simulink model "Computer_Side"  (Simulink 10.0)
settings: Solver=VariableStepAuto  StartTime=0.0  StopTime=inf  FixedStep=1  RelTol=1e-3
undefined symbols (not defined in the file): serial
libraries: instrumentlib x3
settings Model: Creator=fredd  LastModifiedBy=fredd
settings DataIOCC: SaveFormat=Dataset  ReturnWorkspaceOutputs=on
settings OptimizationCC: LifeSpan=auto
settings DebuggingCC: UnderspecifiedInitializationDetection=Simplified  MergeDetectMultiDrivingBlocksExec=error  SFUnexpectedBacktrackingDiag=error  SFNoUnconditionalDefaultTransitionDiag=error  SFExecutionAtInitializationDiag=warning  ArithmeticOperatorsInVariantConditions=error
settings HardwareCC: ProdBitPerPointer=64  ProdBitPerSizeT=64  ProdBitPerPtrDiffT=64  ProdLargestAtomicFloat=Float  ProdIntDivRoundTo=Zero  ProdEndianess=LittleEndian  ProdWordSize=64  ProdHWDeviceType=Intel->x86-64 (Windows64)
settings ModelReferenceCC: PropagateSignalLabelsOutOfModel=on
settings SFSimCC: SimUseLocalCustomCode=on  CustomCodeUndefinedFunction=FilterOut
settings RTWCC: RTWUseLocalCustomCode=on
settings CodeAppCC: StateflowObjectComments=off
settings GRTTargetCC: TargetLangStandard=C99 (ISO)  CombineOutputUpdateFcns=on  GRTInterface=off
settings ConfigComp: CovMetricSettings=dwe  CovHtmlReporting=off  CovSaveCumulativeToWorkspaceVar=off  CovSaveSingleToWorkspaceVar=off

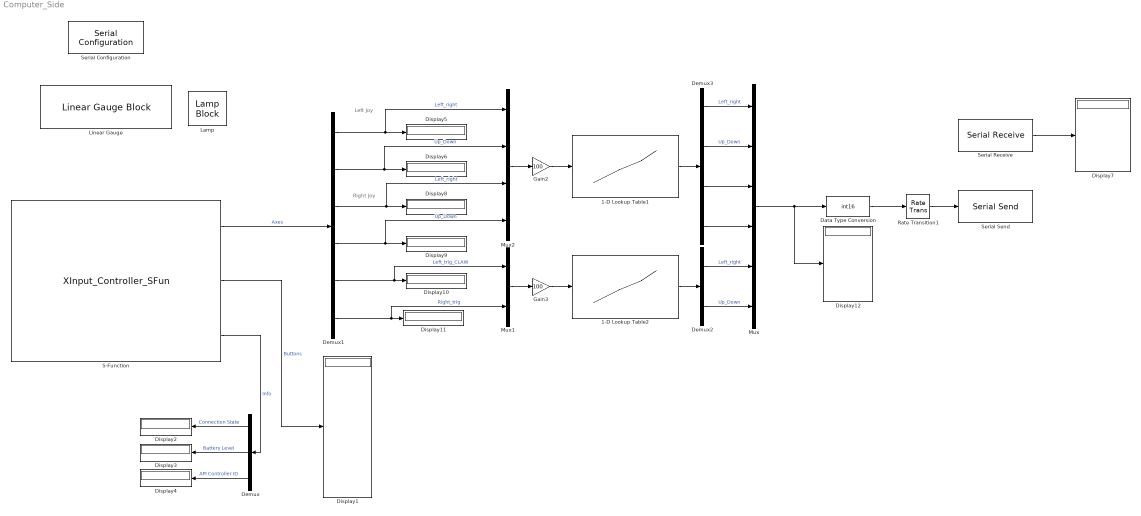
== system Computer_Side ==
  note: Left Joy
  note: Right Joy
  1-D Lookup Table1 : Lookup_n-D  NumberOfTableDimensions=1  BreakpointsForDimension1=[-100,-50,0,50,100]  BreakpointsForDimension1FirstPoint=0  BreakpointsForDimension1Spacing=1.8  Table=[0;45;90;135;180]  InternalRulePriority=Speed  RndMeth=Simplest  InputSameDT=on
  1-D Lookup Table2 : Lookup_n-D  NumberOfTableDimensions=1  BreakpointsForDimension1=[0:5:100]  BreakpointsForDimension1FirstPoint=0  BreakpointsForDimension1Spacing=1.8  Table=[0;9;18;27;36;45;54;63;72;81;90;99;108;117;126;135;144;153;162;171;180]  InternalRulePriority=Speed  RndMeth=Simplest  InputSameDT=on
  Data Type Conversion : DataTypeConversion  OutMin=0  OutMax=100  OutDataTypeStr=int16  RndMeth=Round  SaturateOnIntegerOverflow=on
  Demux : Demux  Outputs=3
  Demux1 : Demux  Outputs=6
  Demux2 : Demux  Outputs=2
  Demux3 : Demux
  Display{1..12} (12 alike) : Display
      Display10 settings: Format=bank  Decimation=2
      Display11 settings: Format=bank  Decimation=2
      Display12 settings: Format=bank  Decimation=2
      Display5 settings: Format=bank  Decimation=2
      Display6 settings: Format=bank  Decimation=2
      Display7 settings: Format=bank  Decimation=2
      Display8 settings: Format=bank  Decimation=2
      Display9 settings: Format=bank  Decimation=2
  Gain2 : Gain  Gain=100
  Gain3 : Gain  Gain=100
  Lamp : LampBlock  DefaultColor=DataTag1  States=DataTag2
  Linear Gauge : LinearGaugeBlock  TickInterval=25  ScaleColors=DataTag4
  Mux : Mux  Inputs=6
  Mux1 : Mux  Inputs=2
  Mux2 : Mux
  Rate Transition1 : RateTransition  OutPortSampleTime=0.01
  S-Function : S-Function  FunctionName=XInput_Controller_SFun  Parameters=ControllerID  SFunctionDeploymentMode=off  EnableBusSupport=off  mask(XInput Controller){ControllerID=1}
      mask help:
      | This Block will allow you to use XInput Controllers in Simulink.
      | XInput is the most Supported API.
      | Works with XBOX 360 and XBOX ONE Controllers.
      |
      | Use 'DEMUX' to access Signals
      | Output_1 [1x6]
      |   Analog Left X, Analog Left Y,
      |   Analog Right X, Analog Right Y,
      |   Left Trigger, Right Trigger
      | Output_2 [1x14]
      |   Up, Down, Left, Right,
      |   Start, Back, Left Stick, Right Stick,
      |   Left Shoulder, Right Shoulder,
      |   A, B, X, Y
      | Output_3 [1x3]
      |   Connection State, Battery Level (1-4), Controller ID
      mask init:
      | ControllerID;   
      | blk = gcb; 
      | get_String = get_param(blk,'ControllerID');
      | ControllerID = str2double(get_String);
      mask Help:
      | Based on Microsoft XInput API
      | Therefore the maximum of conneced Gamepads per PC is 4. First Gamepad has Controller ID 1.
      | 
      | Reference:
      | https://docs.microsoft.com/en-us/windows/win32/api/_xinput/
      | 
      | Tutorial:
      | https://docs.microsoft.com/en-us/windows/win32/xinput/getting-started-with-xinput
      | 
      | Info:
      | The Analog Sticks Deadzone is coded to:
      | Deadzone = 6144;
      | 0 <= Deadzone <= 65534
      | This is smaller then Microsoft default.
      | 
      | created by Mathias Voigt
      | Technische Universität Dresden
      | 2019
      mask TypeOptions ControllerID: 1 | 2 | 3 | 4
      mask Display:
      | %% Set Block picture from user Data
      | %  (permanent, picture file not needed)
      | %  see persistent_image_allocation.m
      | 
      | %get the picture data
      | UserDataStrut = get_param(gcb, 'UserData');
      | image(UserDataStrut.Image, [0.2, 0.3, 0.6, 0.6])
      | 
      | 
      | 
      | % conventional method (does not save picture data in Simulink)
      | % image('XBOX_One_Controller_Icon.png', [0.2, 0.3, 0.6, 0.6])
      | 
      | %% Create Port Labels
      | color('blue');
      | port_label('output', 1, 'Axes');
      | port_label('output', 2, 'Buttons');
      | port_label('output', 3, 'Info');
      | 
      | 
      | %% Create S-Function Block Name
      | color('black');
      | text(0.5, 0.1, 'XInput Controller',...
      |      'horizontalAlignment', 'center',...
      |      'verticalAlignment', 'bottom');
  Serial Configuration : instrumentlib/Serial Configuration  Priority=-200000  ComPortMenu=COM3  ComPort=COM3  ObjConstructor=serial('COM3');  BaudRate=57600  DataBits=8  Parity=none  StopBits=1  FlowControl=none  Timeout=10  ByteOrder=LittleEndian
  Serial Receive : instrumentlib/Serial Receive  ComPortMenu=COM3  ComPort=COM3  ObjConstructor=serial('COM3');  Terminator=<none>  DataSize=6  DataType=int16  EnableBlockingMode=on  ActionDataUnavailable=Output last received value  CustomValue=0  SampleTime=0.01
  Serial Send : instrumentlib/Serial Send  ComPortMenu=COM3  ComPort=COM3  ObjConstructor=serial('COM3');  Terminator=<none>  EnableBlockingMode=off
  wires:
  Serial Receive/1 -> Display7/1
  Data Type Conversion/1 -> Rate Transition1/1
  Rate Transition1/1 -> Serial Send/1
  Demux/3 -> Display4/1  "API Controller ID"
  S-Function/3 -> Demux/1  "Info"
  Demux/1 -> Display2/1  "Connection State"
  Demux/2 -> Display3/1  "Battery Level"
  S-Function/2 -> Display1/1  "Buttons"
  S-Function/1 -> Demux1/1  "Axes"
  Demux1/2 -> Mux2/2, Display6/1  "Up_Down"
  Demux1/3 -> Mux2/3, Display8/1  "Left_right"
  Demux1/4 -> Mux2/4, Display9/1  "Up_Down"
  Demux1/5 -> Mux1/1, Display10/1  "Left_trig_CLAW"
  Demux1/6 -> Mux1/2, Display11/1  "Right_trig"
  Demux1/1 -> Mux2/1, Display5/1  "Left_right"
  Mux/1 -> Data Type Conversion/1, Display12/1
  Mux1/1 -> Gain3/1
  1-D Lookup Table2/1 -> Demux2/1
  Demux2/1 -> Mux/5  "Left_right"
  Demux2/2 -> Mux/6  "Up_Down"
  Mux2/1 -> Gain2/1
  1-D Lookup Table1/1 -> Demux3/1
  Demux3/1 -> Mux/1  "Left_right"
  Demux3/2 -> Mux/2  "Up_Down"
  Demux3/3 -> Mux/3
  Demux3/4 -> Mux/4
  Gain2/1 -> 1-D Lookup Table1/1
  Gain3/1 -> 1-D Lookup Table2/1
